simulink model "example_Fuel"  (R2013b)
settings: Solver=ode45  StartTime=0.0  StopTime=10.0  RelTol=1e-3
libraries: carnot x4
settings Model: Creator=drhf  LastModifiedBy=drhf
settings OptimizationCC: InlineParams=on

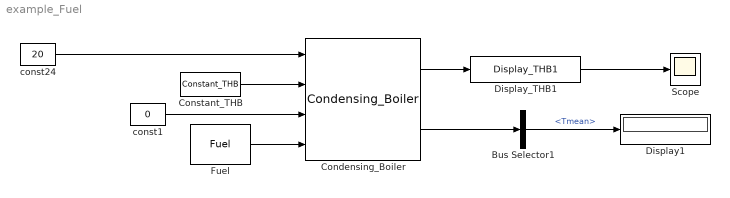
== system example_Fuel ==
  Bus Selector1 : BusSelector  OutputSignals=Tmean
  Condensing_Boiler : carnot/Source/Boiler/Condensing_Boiler  Pnom=20e3  U=3  vol=0.02  relativeQdot=[0.25 1]  temperatures="[40  70]"  efficiency=[1.05 0.95; 1.0 0.9]  electricPower=[20 120]  lin=10  qua=100  Tini=20  nodes=1
  Constant_THB : carnot/Source/Simple/Constant_THB  t=40  mdot=0  p=1e5  mID=No Pressure Drop  fluid=Water  mix=0  dia=0.02  hgt=0
  Display1 : Display
  Display_THB1 : carnot/Outputs/Display_THB1  t=on  m=off  p=off  id=off  mix=off  d=off
  Fuel : carnot/Source/Energy/Fuel  ft=1  t=20  ls=1  p=1e5  h_values=[5.14e7 5.69e7]  tc=45  price=1  mass=[0.33 0.67 0 0 0 0]
  Scope : Scope
  const1 : Constant  Value=0
  const24 : Constant  Value=20
  wires:
  Fuel/1 -> Condensing_Boiler/4
  Constant_THB/1 -> Condensing_Boiler/2
  const24/1 -> Condensing_Boiler/1
  const1/1 -> Condensing_Boiler/3
  Condensing_Boiler/1 -> Display_THB1/1
  Display_THB1/1 -> Scope/1
  Condensing_Boiler/2 -> Bus Selector1/1
  Bus Selector1/1 -> Display1/1  "<Tmean>"
